simulink model "blockdemo"  (Simulink 7.3)
settings: Solver=VariableStepDiscrete  StartTime=0.0  StopTime=200  MaxStep=1  RelTol=1e-3
InitFcn:
  | %% DSPBuilder Start
  | alt_dspbuilder_update_model(bdroot)
  | %% DSPBuilder End
libraries: allblocks_alteradspbuilder2 x14, simulink x1
settings Model: Creator=cpurcell  LastModifiedBy=dyfong
settings OptimizationCC: InitFltsAndDblsToZero=on
settings DebuggingCC: SaveWithParameterizedLinksMsg=none  SignalResolutionControl=TryResolveAllWithWarning  MultiTaskCondExecSysMsg=none
settings RTWCC: IncludeERTFirstTime=on
settings GRTTargetCC: TargetFcnLib=ansi_tfl_tmw.mat

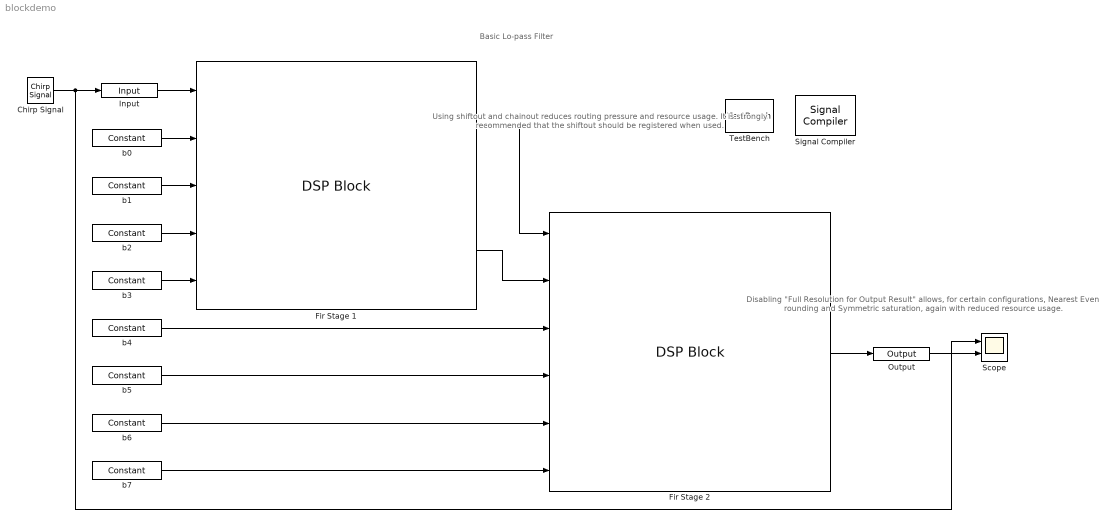
== system blockdemo ==
  note: Basic Lo-pass Filter
  note: Using shiftout and chainout
      | reduces routing pressure
      | and resource usage. It is strongly
      | recommended that the shiftout
      | should be registered when used.
  note: Disabling "Full Resolution for Output
      | Result" allows, for certain configurations,
      | Nearest Even rounding and Symmetric
      | saturation, again with reduced resource
      | usage.
  Chirp Signal : simulink/Sources/Chirp Signal  SystemSampleTime=-1  f1=0.1  T=100  f2=1
  Fir Stage 1 : allblocks_alteradspbuilder2/DSP Block  multipliers=4  BusType=Signed Fractional  bwlA=2  bwrA=16  inputWidthACalc=18  bwlB=0  bwrB=18  inputWidthBCalc=18  shift_mode=on  use_shiftout=on  mult1_direction=ADD  mult3_direction=ADD  accumulator=off  accum_direction=ADD  use_accum_sload=off  okForChainoutCalc=1  chainout_adder=off  use_chainout=on  use_zero_chainout=off  full_resolution=off  bwlOutfix=10  bwrOutfix=34  bwrMultCalc=34  bwlMultCalc=10  bwrOutCalc=34  bwlOutCalc=10  outputWidthCalc=44  output_msb=44  single_dsp_block=1  support_rounding_saturation=1  output_lsb=0  width_msb=44  output_rounding_possible=0  output_round_type=None (truncate)  output_rounding=0  width_saturate_sign=0  output_saturation_possible=0  output_saturate_type=None (wrap)  output_saturation=0  use_overflow=off  port_output_is_overflow=0  register_data_inputs=off  register_multiplier=on  register_adder=on  reg_chainout=on  reg_shiftout=on  model_is_delayed=1  use_ena=off  use_aclr=off  pipeline_display=2
  Fir Stage 2 : allblocks_alteradspbuilder2/DSP Block  multipliers=4  BusType=Signed Fractional  bwlA=2  bwrA=16  inputWidthACalc=18  bwlB=0  bwrB=18  inputWidthBCalc=18  shift_mode=on  use_shiftout=off  mult1_direction=ADD  mult3_direction=ADD  accumulator=off  accum_direction=ADD  use_accum_sload=off  okForChainoutCalc=1  chainout_adder=on  use_chainout=off  use_zero_chainout=off  full_resolution=off  bwlOutfix=1  bwrOutfix=16  bwrMultCalc=34  bwlMultCalc=10  bwrOutCalc=16  bwlOutCalc=1  outputWidthCalc=17  output_msb=35  single_dsp_block=1  support_rounding_saturation=1  output_lsb=18  width_msb=17  output_rounding_possible=1  output_round_type=Nearest Even  output_rounding=1  width_saturate_sign=9  output_saturation_possible=1  output_saturate_type=Symmetric  output_saturation=1  use_overflow=off  port_output_is_overflow=0  register_data_inputs=off  register_multiplier=on  register_adder=on  reg_chainout=on  reg_shiftout=on  model_is_delayed=1  use_ena=off  use_aclr=off  pipeline_display=2
  Input : allblocks_alteradspbuilder2/Input  iofile=/data/dyfong/qshell/110_64/p4/dsp_builder/dsp_builder2/Documentation/DesignExamples/Tutorials/UnitBlocks/Arithmetic/MultiplyAddStratixIII/tb_blockdemo/blockdemo_Input.salt  BusType=Signed Fractional  bwl=2  bwr=16  SpecifyClock=off  PORTTYPE=Input  externalType=Inferred  allowFloatingPointOverride=on  logOutputs=off
  Output : allblocks_alteradspbuilder2/Output  iofile=/data/dyfong/qshell/110_64/p4/dsp_builder/dsp_builder2/Documentation/DesignExamples/Tutorials/UnitBlocks/Arithmetic/MultiplyAddStratixIII/tb_blockdemo/blockdemo_Output.capture  BusType=Signed Fractional  bwl=2  bwr=16  externalType=Inferred  PORTTYPE=Output  allowFloatingPointOverride=on  logOutputs=off
  Scope : Scope  NumInputPorts=2
      settings: TimeRange=200  YMin=-1~-1  YMax=1~1
  Signal Compiler : allblocks_alteradspbuilder2/Signal Compiler  DeviceFamily=Stratix III  DeviceName=AUTO  EnableSignalTap=off  SignalTapDepth=128  UseBoardBlock=off  StpUseDefaultClock=on  StpClock=Clock  ExportDir=D:\
  TestBench : allblocks_alteradspbuilder2/TestBench  enable=on  advancedMode=off  modelSimGui=off  maxDisplayErrors=10  mismatchErrorLevel=Error  simdatafile=/data/dyfong/qshell/110_64/p4/dsp_builder/dsp_builder2/Documentation/DesignExamples/Tutorials/UnitBlocks/Arithmetic/MultiplyAddStratixIII/tb_blockdemo/blockdemo.simdata.tcl
  b0 : allblocks_alteradspbuilder2/Constant  mask_cst=-0.0863083  BusType=Signed Fractional  bwl=0  bwr=18  roundMode=Truncate  satMode=Wrap  SpecifyClock=off  allowFloatingPointOverride=on  logOutputs=off  logFile=/data/dyfong/qshell/110_64/p4/dsp_builder/dsp_builder2/Documentation/DesignExamples/Tutorials/UnitBlocks/Arithmetic/MultiplyAddStratixIII/tb_blockdemo/blockdemo_b0.fixedpointlog
  b1 : allblocks_alteradspbuilder2/Constant  mask_cst=5.85944E-4  BusType=Signed Fractional  bwl=0  bwr=18  roundMode=Truncate  satMode=Wrap  SpecifyClock=off  allowFloatingPointOverride=on  logOutputs=off  logFile=/data/dyfong/qshell/110_64/p4/dsp_builder/dsp_builder2/Documentation/DesignExamples/Tutorials/UnitBlocks/Arithmetic/MultiplyAddStratixIII/tb_blockdemo/blockdemo_b1.fixedpointlog
  b2 : allblocks_alteradspbuilder2/Constant  mask_cst=0.201995  BusType=Signed Fractional  bwl=0  bwr=18  roundMode=Truncate  satMode=Wrap  SpecifyClock=off  allowFloatingPointOverride=on  logOutputs=off  logFile=/data/dyfong/qshell/110_64/p4/dsp_builder/dsp_builder2/Documentation/DesignExamples/Tutorials/UnitBlocks/Arithmetic/MultiplyAddStratixIII/tb_blockdemo/blockdemo_b2.fixedpointlog
  b3 : allblocks_alteradspbuilder2/Constant  mask_cst=0.373711  BusType=Signed Fractional  bwl=0  bwr=18  roundMode=Truncate  satMode=Wrap  SpecifyClock=off  allowFloatingPointOverride=on  logOutputs=off  logFile=/data/dyfong/qshell/110_64/p4/dsp_builder/dsp_builder2/Documentation/DesignExamples/Tutorials/UnitBlocks/Arithmetic/MultiplyAddStratixIII/tb_blockdemo/blockdemo_b3.fixedpointlog
  b4 : allblocks_alteradspbuilder2/Constant  mask_cst=0.373711  BusType=Signed Fractional  bwl=0  bwr=18  roundMode=Truncate  satMode=Wrap  SpecifyClock=off  allowFloatingPointOverride=on  logOutputs=off  logFile=/data/dyfong/qshell/110_64/p4/dsp_builder/dsp_builder2/Documentation/DesignExamples/Tutorials/UnitBlocks/Arithmetic/MultiplyAddStratixIII/tb_blockdemo/blockdemo_b4.fixedpointlog
  b5 : allblocks_alteradspbuilder2/Constant  mask_cst=0.201995  BusType=Signed Fractional  bwl=0  bwr=18  roundMode=Truncate  satMode=Wrap  SpecifyClock=off  allowFloatingPointOverride=on  logOutputs=off  logFile=/data/dyfong/qshell/110_64/p4/dsp_builder/dsp_builder2/Documentation/DesignExamples/Tutorials/UnitBlocks/Arithmetic/MultiplyAddStratixIII/tb_blockdemo/blockdemo_b5.fixedpointlog
  b6 : allblocks_alteradspbuilder2/Constant  mask_cst=5.85944E-4  BusType=Signed Fractional  bwl=0  bwr=18  roundMode=Truncate  satMode=Wrap  SpecifyClock=off  allowFloatingPointOverride=on  logOutputs=off  logFile=/data/dyfong/qshell/110_64/p4/dsp_builder/dsp_builder2/Documentation/DesignExamples/Tutorials/UnitBlocks/Arithmetic/MultiplyAddStratixIII/tb_blockdemo/blockdemo_b6.fixedpointlog
  b7 : allblocks_alteradspbuilder2/Constant  mask_cst=-0.0863083  BusType=Signed Fractional  bwl=0  bwr=18  roundMode=Truncate  satMode=Wrap  SpecifyClock=off  allowFloatingPointOverride=on  logOutputs=off  logFile=/blockdemo_b7.fixedpointlog
  wires:
  b3/1 -> Fir Stage 1/5
  b2/1 -> Fir Stage 1/4
  b1/1 -> Fir Stage 1/3
  b0/1 -> Fir Stage 1/2
  Input/1 -> Fir Stage 1/1
  b7/1 -> Fir Stage 2/6
  b6/1 -> Fir Stage 2/5
  b5/1 -> Fir Stage 2/4
  b4/1 -> Fir Stage 2/3
  Fir Stage 1/2 -> Fir Stage 2/2
  Fir Stage 1/1 -> Fir Stage 2/1
  Fir Stage 2/1 -> Output/1
  Chirp Signal/1 -> Input/1, Scope/1
  Output/1 -> Scope/2
